simulink model "PIDSystem"  (R2024b)
settings: Solver=VariableStepAuto  StartTime=0.0  StopTime=10.0  RelTol=1e-3
values from neighbouring files (symbols this model uses):
  disorder_times = [10, 14]    [assignment1.m]
  sys = sys(end)    [assignment1.m]
  u_control = 0.5    [assignment1.m]
  z = 0.1    [assignment1.m]
undefined symbols (not defined in the file or in its folder): DC, IC, PC
settings Model: Creator=lukiq  LastModifiedBy=lukiq

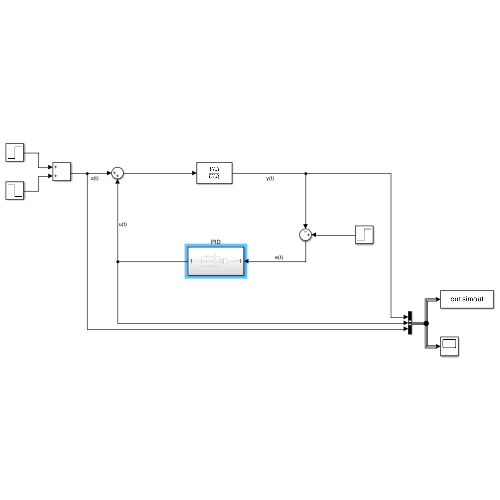
[thumbnail: Simulink's stored preview of the top-level diagram]
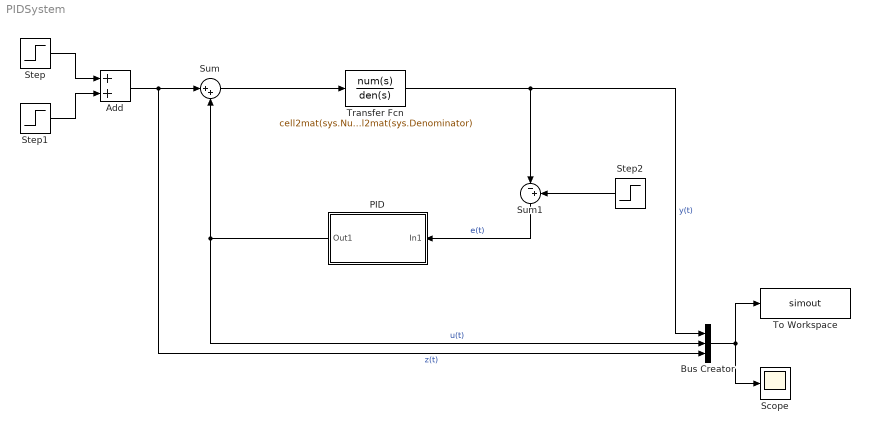
== system PIDSystem ==
  Add : Sum
  Bus Creator : BusCreator  Inputs=3
  PID : Subsystem
  Scope : Scope
  Step : Step  Time=disorder_times(1)  After=z * u_control  SampleTime=0
  Step1 : Step  Time=disorder_times(2)  After=-z * u_control  SampleTime=0
  Step2 : Step  Time=0  After=u_control  SampleTime=0
  Sum : Sum  Inputs=|++
  Sum1 : Sum  Inputs=|-+
  To Workspace : ToWorkspace  VariableName=simout  SaveFormat=Timeseries  SampleTime=-1
  Transfer Fcn : TransferFcn  Numerator=cell2mat(sys.Numerator)  Denominator=cell2mat(sys.Denominator)
  wires:
  Sum/1 -> Transfer Fcn/1
  PID/1(Out1) -> Bus Creator/2, Sum/2  "u(t)"
  Add/1 -> Bus Creator/3, Sum/1  "z(t)"
  Step/1 -> Add/1
  Step1/1 -> Add/2
  Sum1/1 -> PID/1(In1)  "e(t)"
  Transfer Fcn/1 -> Bus Creator/1, Sum1/1  "y(t)"
  Step2/1 -> Sum1/2
  Bus Creator/1 -> Scope/1, To Workspace/1

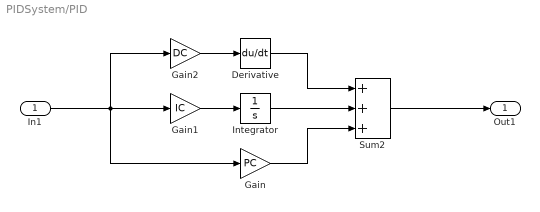
== system PIDSystem/PID ==
  In1 : Inport
  Derivative : Derivative
  Gain : Gain  Gain=PC
  Gain1 : Gain  Gain=IC
  Gain2 : Gain  Gain=DC
  Integrator : Integrator
  Sum2 : Sum  Inputs=+++
  Out1 : Outport
  wires:
  Derivative/1 -> Sum2/1
  Integrator/1 -> Sum2/2
  Gain/1 -> Sum2/3
  In1/1 -> Gain1/1, Gain/1, Gain2/1
  Gain1/1 -> Integrator/1
  Gain2/1 -> Derivative/1
  Sum2/1 -> Out1/1
